simulink model "operational_space_inv_dyn"  (R2020b)
settings: Solver=FixedStepAuto  StartTime=0.0  StopTime=10  FixedStep=Ts  RelTol=1e-3
undefined symbols (not defined in the file): dqi, he, KD, KP, myRobot, qi, xf, xi
libraries: vrlib x1
settings Model: Creator=simon  LastModifiedBy=SimoneCremasco
settings SolverCC: ZeroCrossControl=DisableAll

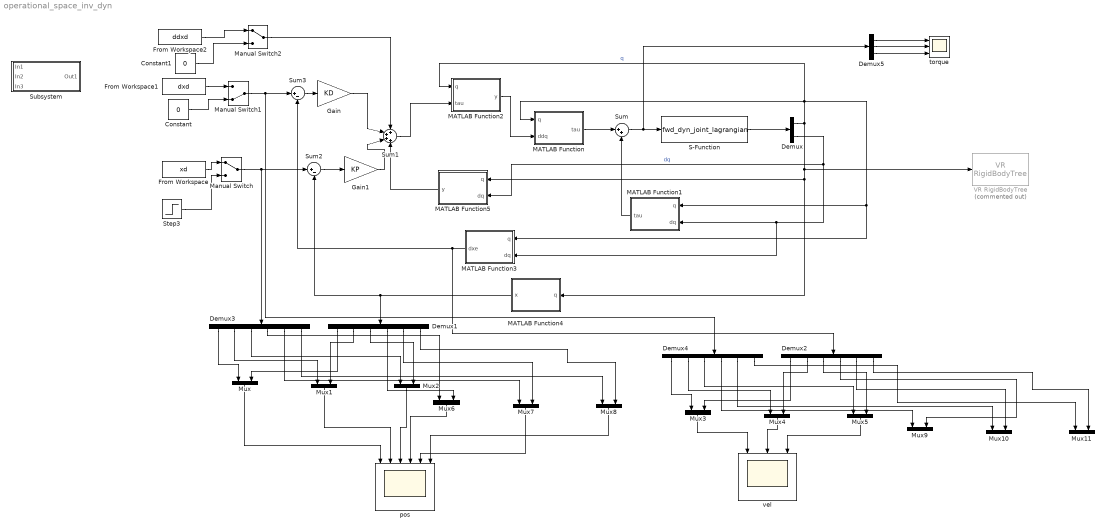
== system operational_space_inv_dyn ==
  Constant : Constant  Value=0
  Constant1 : Constant  Value=0
  Demux : Demux  Outputs=2
  Demux{1..4} (4 alike) : Demux  Outputs=6
  Demux5 : Demux  Outputs=3
  From Workspace : FromWorkspace  VariableName=xd
  From Workspace1 : FromWorkspace  VariableName=dxd
  From Workspace2 : FromWorkspace  VariableName=ddxd
  Gain : Gain  Gain=KD
  Gain1 : Gain  Gain=KP
  MATLAB Function : MATLAB Function  TreatAsAtomicUnit=on
  MATLAB Function1 : MATLAB Function  TreatAsAtomicUnit=on
  MATLAB Function2 : MATLAB Function  TreatAsAtomicUnit=on
  MATLAB Function3 : MATLAB Function  TreatAsAtomicUnit=on
  MATLAB Function4 : MATLAB Function  TreatAsAtomicUnit=on
  MATLAB Function5 : MATLAB Function  TreatAsAtomicUnit=on
  Manual Switch : ManualSwitch
  Manual Switch1 : ManualSwitch  CurrentSetting=0
  Manual Switch2 : ManualSwitch
  Mux{,1..11} (12 alike) : Mux  Inputs=2
  S-Function : S-Function  FunctionName=fwd_dyn_joint_lagrangian  Parameters=myRobot,he,qi,dqi  SFunctionDeploymentMode=off  EnableBusSupport=off
  Step3 : Step  Before=xi  After=xf  SampleTime=0
  Subsystem : Subsystem
  Sum : Sum  Inputs=|++
  Sum1 : Sum  Inputs=++++
  Sum2 : Sum  Inputs=|+-
  Sum3 : Sum  Inputs=|+-
  VR RigidBodyTree : vrlib/VR RigidBodyTree  Commented=on  RBT=rbt  useRBT=on  Ts=-1  ForceViewerOpen=on
      settings: SourceProductBaseCode=SL
  pos : Scope  NumInputPorts=6
  torque : Scope  NumInputPorts=3
  vel : Scope  NumInputPorts=3
  wires:
  S-Function/1 -> Demux/1
  MATLAB Function/1(tau) -> Sum/1
  MATLAB Function1/1(tau) -> Sum/2
  Sum/1 -> Demux5/1, S-Function/1
  Gain1/1 -> Sum1/3
  Gain/1 -> Sum1/2
  Sum3/1 -> Gain/1
  Sum2/1 -> Gain1/1
  Mux1/1 -> pos/2
  Mux2/1 -> pos/3
  Demux1/3 -> Mux2/2
  Mux/1 -> pos/1
  Demux1/2 -> Mux1/2
  Demux1/1 -> Mux/2
  Demux3/1 -> Mux/1
  Demux/1 -> VR RigidBodyTree/1, MATLAB Function5/1(q), MATLAB Function4/1(q), MATLAB Function3/1(q), MATLAB Function1/1(q), MATLAB Function2/1(q), MATLAB Function/1(q)  "q"
  Demux3/2 -> Mux1/1
  Demux3/3 -> Mux2/1
  Demux/2 -> MATLAB Function5/2(dq), MATLAB Function3/2(dq), MATLAB Function1/2(dq)  "dq"
  Demux4/2 -> Mux4/1
  Demux4/3 -> Mux5/1
  Demux4/1 -> Mux3/1
  Mux5/1 -> vel/3
  Mux3/1 -> vel/1
  Demux2/3 -> Mux5/2
  Mux4/1 -> vel/2
  Demux2/1 -> Mux3/2
  Demux2/2 -> Mux4/2
  MATLAB Function2/1(y) -> MATLAB Function/2(ddq)
  Sum1/1 -> MATLAB Function2/2(tau)
  MATLAB Function3/1(dxe) -> Sum3/2, Demux2/1
  MATLAB Function4/1(x) -> Demux1/1, Sum2/2
  MATLAB Function5/1(y) -> Sum1/4
  Demux3/4 -> Mux6/1
  Demux3/6 -> Mux8/1
  Demux3/5 -> Mux7/1
  Demux1/4 -> Mux6/2
  Demux1/6 -> Mux8/2
  Demux1/5 -> Mux7/2
  Demux4/5 -> Mux10/1
  Demux2/4 -> Mux9/2
  Demux2/5 -> Mux10/2
  Demux4/6 -> Mux11/1
  Demux2/6 -> Mux11/2
  Demux4/4 -> Mux9/1
  Manual Switch/1 -> Demux3/1, Sum2/1
  From Workspace/1 -> Manual Switch/1
  Step3/1 -> Manual Switch/2
  Manual Switch1/1 -> Demux4/1, Sum3/1
  From Workspace1/1 -> Manual Switch1/1
  Constant/1 -> Manual Switch1/2
  Manual Switch2/1 -> Sum1/1
  From Workspace2/1 -> Manual Switch2/1
  Constant1/1 -> Manual Switch2/2
  Demux5/1 -> torque/1
  Demux5/2 -> torque/2
  Demux5/3 -> torque/3
  Mux6/1 -> pos/4
  Mux7/1 -> pos/5
  Mux8/1 -> pos/6

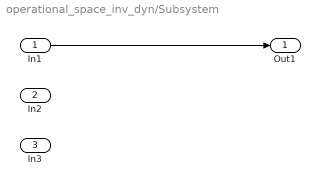
== system operational_space_inv_dyn/Subsystem ==
  In1 : Inport
  In2 : Inport  Port=2
  In3 : Inport  Port=3
  Out1 : Outport
  wires:
  In1/1 -> Out1/1

== matlab function operational_space_inv_dyn/MATLAB Function ==
  data: q input size=3; tau output; ddq input size=3
function tau = B(q, ddq)

tau = getB(q)*ddq;

== matlab function operational_space_inv_dyn/MATLAB Function2 ==
  data: q input; y output; tau input
function y = invJa(q, tau)

y = getInvJa(q)*tau;

== matlab function operational_space_inv_dyn/MATLAB Function3 ==
  data: q input; dxe output; dq input
function dxe = Ja(q, dq)

dxe = getJa(q)*dq;

== matlab function operational_space_inv_dyn/MATLAB Function4 ==
  data: q input; x output
function x = k(q)

x = getK(q);

== matlab function operational_space_inv_dyn/MATLAB Function5 ==
  data: q input; y output; dq input
function y = dJa(q, dq)

y = getDiffJa(q)*dq;

== matlab function operational_space_inv_dyn/MATLAB Function1 ==
  data: q input size=3; tau output; dq input size=3
function tau = n(q, dq)

tau = getN(q, dq);
